simulink model "DemoUSRPTXBernoulli"  (Simulink 7.7)
settings: Solver=ode45  StartTime=0.0  StopTime=10  RelTol=1e-3
PreLoadFcn:
  | EbNo = 16; Errors = 188; Bits = 1e8; M = 256; N = 64; Ts = (1/22050); constellation; InnerInterleaverBitTable
undefined symbols (not defined in the file or in its folder): rsgenpoly
libraries: dspmtrx3 x16, simulink x9, commutil2 x3, commrandsrc2 x2, commblkintrlv2 x2, commblkcod2 x1, dspindex x1, commseqgen2 x1, commcnvintrlv2 x1, commcnvcod2 x1, dspxfrm3 x1, dspsigops x1
settings Model: Creator=katsikas  LastModifiedBy=katsikas
settings SimEventsCC: propDiagAttribOutput=1  propDiagFcnCallOutput=1  propDiagStatOutput=0

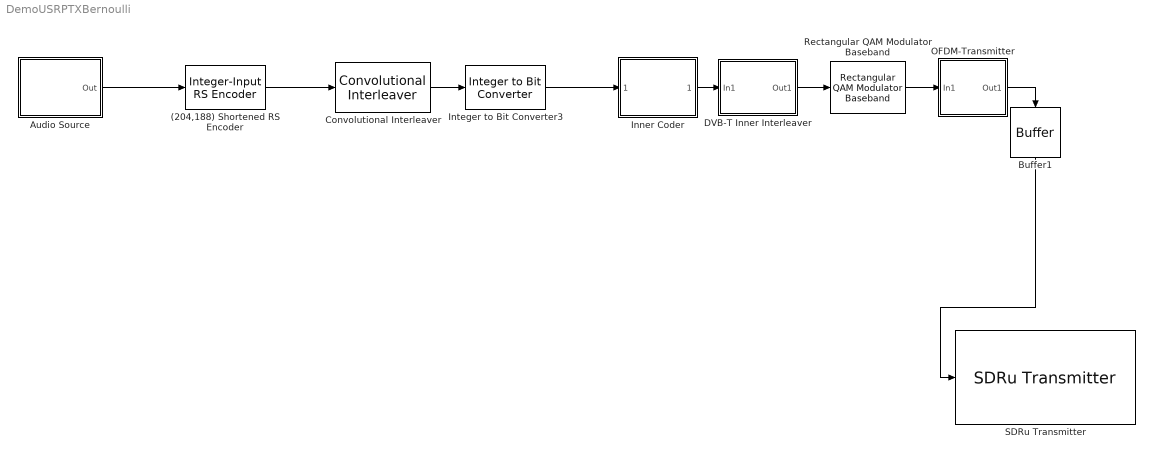
== system DemoUSRPTXBernoulli ==
  (204,188) Shortened RS Encoder : commblkcod2/Integer-Input RS Encoder  n=204  k=188  specPrimPoly=off  prPoly=[1 0 1 1]  specGenPoly=off  genPoly=rsgenpoly(7,3)  specPuncture=off  punctVec=[ones(2,1); zeros(2,1)]
  Audio Source : Subsystem
  Buffer1 : Buffer  N=2048  TreatMby1Signals=One channel
  Convolutional Interleaver : commcnvintrlv2/Convolutional Interleaver  SystemSampleTime=-1  N=12  B=17  ic=0
  DVB-T Inner Interleaver : Subsystem  mask(DVB-T Inner Interleaver){}
      mask init:
      | fullILVec = [(1:126) ...
      |  (rem([0:125]+63,126) +1 + 126     ) ...
      |  (rem([0:125]+105,126)+1 + (2*126) ) ...
      |  (rem([0:125]+42,126) +1 + (3*126) ) ...
      |  (rem([0:125]+21,126) +1 + (4*126) ) ...
      |  (rem([0:125]+84,126) +1 + (5*126) )];
      mask Display: disp('DVB-T\nInner\nInterleaver')
  Inner Coder : Subsystem
      mask Display: disp('Rate 3/4\nPunctured\nConvolutional\nCode');
  Integer to Bit Converter3 : commutil2/Integer to Bit Converter  nbits=log2(M)  signedInputValues=Unsigned  bitOrder=MSB first  outDtype=boolean
  OFDM-Transmitter : Subsystem
  Rectangular QAM Modulator Baseband : commdigbbndam3/Rectangular QAM Modulator Baseband  M=N  InType=Bit  Enc=User-defined  Mapping=map_constellation  PowType=Average Power  MinDist=2  AvgPow=1  PeakPow=1  Ph=0  outDtype=double  outWordLen=16  outUDDataType=sfix(16)  outFracLenMode=Best precision  outFracLen=15
  SDRu Transmitter : commsdrhw_v2/SDRu Transmitter  SystemSampleTime=-1  rxtx=tx  USRP2_IP='192.168.10.2'  centerFrequency=482e6  centerFrequencySrc=Dialog  loOffset=0  loOffsetSrc=Dialog  gain=20  gainSrc=Dialog  decimInterp=512  decimInterpSrc=Dialog  USRP2_IP_NUM=[49 57 50 46 49 54 56 46 49 48 46 50]  frameLength=362  outputDatatype=int16  overrunUnderrunPort=off  sampleTime=1  dboardInfo=|  HOST_DATA_PORT=30000  HOST_CONTROL_PORT=30001  USRP2_DATA_PORT=32769  USRP2_CONTROL_PORT=32768
      | dbid: 0
      |           dbName: 'no db found'
      |          freqMin: 0
      |          freqMax: 0
      |          gainMin: 0
      |          gainMax: 0
      |     gainStepSize: 0
  wires:
  Rectangular QAM Modulator Baseband/1 -> OFDM-Transmitter/1(In1)
  Convolutional Interleaver/1 -> Integer to Bit Converter3/1
  (204,188) Shortened RS Encoder/1 -> Convolutional Interleaver/1
  Integer to Bit Converter3/1 -> Inner Coder/1(Uncoded symbols)
  Inner Coder/1(Coded bits) -> DVB-T Inner Interleaver/1(In1)
  DVB-T Inner Interleaver/1(Out1) -> Rectangular QAM Modulator Baseband/1
  Audio Source/1(Out) -> (204,188) Shortened RS Encoder/1
  OFDM-Transmitter/1(Out1) -> Buffer1/1
  Buffer1/1 -> SDRu Transmitter/1

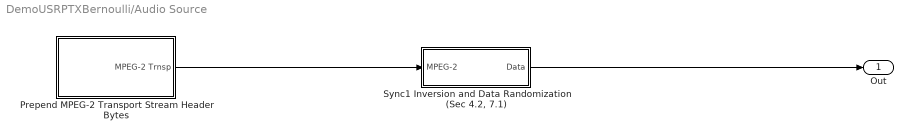
== system DemoUSRPTXBernoulli/Audio Source ==
  Prepend MPEG-2 Transport Stream Header Bytes : Subsystem
      mask Display: disp(sprintf('Prepend MPEG-2\nTransportStream\nHeader Bytes'))
  "Sync1 Inversion and Data Randomization (Sec 4.2, 7.1)" : Subsystem
  Out : Outport
  wires:
  Prepend MPEG-2 Transport Stream Header Bytes/1(MPEG-2 Trnsp) -> "Sync1 Inversion and Data Randomization (Sec 4.2, 7.1)"/1(MPEG-2)
  "Sync1 Inversion and Data Randomization (Sec 4.2, 7.1)"/1(Data) -> Out/1

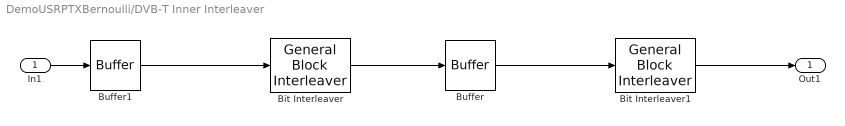
== system DemoUSRPTXBernoulli/DVB-T Inner Interleaver ==
  In1 : Inport
  Bit Interleaver : commblkintrlv2/General Block Interleaver  elements=BitInterleaverTable
  Bit Interleaver1 : commblkintrlv2/General Block Interleaver  elements=SymbolInterleaverTable
  Buffer : Buffer  N=9072  TreatMby1Signals=One channel
  Buffer1 : Buffer  N=756  TreatMby1Signals=One channel
  Out1 : Outport
  wires:
  In1/1 -> Buffer1/1
  Buffer/1 -> Bit Interleaver1/1
  Buffer1/1 -> Bit Interleaver/1
  Bit Interleaver/1 -> Buffer/1
  Bit Interleaver1/1 -> Out1/1

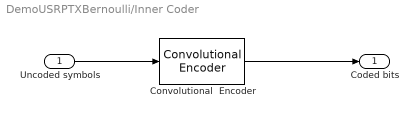
== system DemoUSRPTXBernoulli/Inner Coder ==
  Uncoded symbols : Inport
  Convolutional  Encoder : commcnvcod2/Convolutional Encoder  trellis=poly2trellis(7, [171 133])  opMode=Continuous  DelayedResetAction=off  hasIniStPort=off  hasFinStPort=off  usePuncVector=on  punctureVector=[1 1 0 1 1 0]'  reset=Unused parameter value
  Coded bits : Outport
  wires:
  Convolutional  Encoder/1 -> Coded bits/1
  Uncoded symbols/1 -> Convolutional  Encoder/1

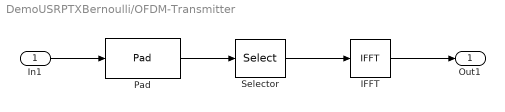
== system DemoUSRPTXBernoulli/OFDM-Transmitter ==
  In1 : Inport
  IFFT : dspxfrm3/IFFT  CompMethod=Table lookup  TableOpt=NEW  TableOptActive=Speed  BitRevOrder=off  cs_in=off  SkipNorm=on  InheritFFTLength=on  FFTLength=64  mode=Complex  outSamplingMode=Frame based  RowConvenienceOn=on  firstCoeffDataTypeStr=Inherit: Same word length as input  firstCoeffLastDataTypeStr=Inherit: Same word length as input  outputMin=[]  outputMax=[]  roundingMode=Floor  overflowMode=off
  Pad : dspsigops/Pad  padAlong=Columns  dimsToPad=1  valSrc=Specify via dialog  padVal=0  spec=Output size  padNumOutRowsSpecMethod=User-specified  numOutRows=2048  padNumOutColsSpecMethod=User-specified  numOutCols=1  isVarDimsMode=off  padBeginning=0  padEnd=0  outSizeMode=User-specified  outSize=1  padSigAt=End  trunc_flag=None  roundingMode=Floor  overflowMode=off  truncOrWrapMode=Truncate  wrap_flag=None
  Selector : Selector  NumberOfDimensions=2  InputPortWidth=3  IndexOptions=Index vector (dialog),Select all  Indices=[1:756 1513:2048 757:1512],1  OutputSizes=1,1
  Out1 : Outport
  wires:
  Pad/1 -> Selector/1
  Selector/1 -> IFFT/1
  IFFT/1 -> Out1/1
  In1/1 -> Pad/1

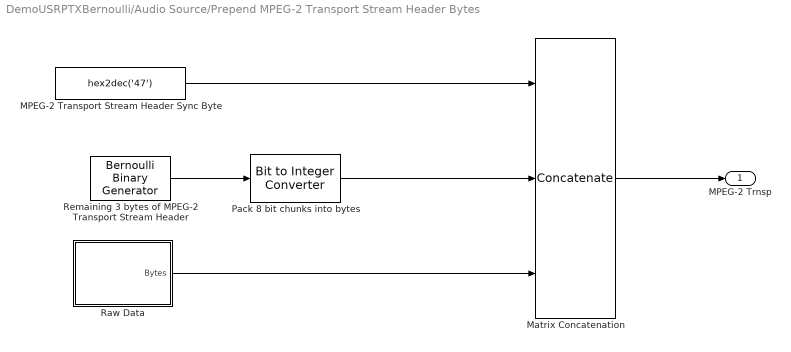
== system DemoUSRPTXBernoulli/Audio Source/Prepend MPEG-2 Transport Stream Header Bytes ==
  MPEG-2 Transport Stream Header Sync Byte : Constant  Value=hex2dec('47')  VectorParams1D=off  OutDataTypeStr=uint8  FramePeriod=(8*188)/9.6e6
      settings: SamplingMode=Frame based
  Matrix Concatenation : Concatenate  NumInputs=3  Mode=Multidimensional array
  Pack 8 bit chunks into bytes : commutil2/Bit to Integer Converter  nbits=8  bitOrder=MSB first  signedOutputValues=Unsigned  outDtype=uint8  outDtypeSigned=Inherit via internal rule
  "Raw Data " : Subsystem
  Remaining 3 bytes of MPEG-2 Transport Stream Header : commrandsrc2/Bernoulli Binary Generator  SystemSampleTime=-1  P=0.5  seed=61  Ts=(8*188/9.6e6) / (3*8)  frameBased=on  sampPerFrame=3*8  orient=off  outDataType=uint8
  MPEG-2 Trnsp : Outport
  wires:
  MPEG-2 Transport Stream Header Sync Byte/1 -> Matrix Concatenation/1
  Remaining 3 bytes of MPEG-2 Transport Stream Header/1 -> Pack 8 bit chunks into bytes/1
  Matrix Concatenation/1 -> MPEG-2 Trnsp/1
  Pack 8 bit chunks into bytes/1 -> Matrix Concatenation/2
  "Raw Data "/1(Bytes) -> Matrix Concatenation/3

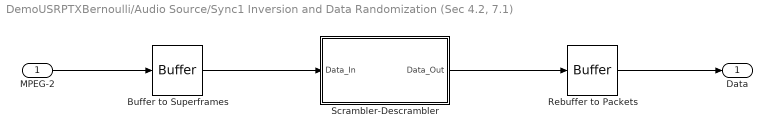
== system DemoUSRPTXBernoulli/Audio Source/Sync1 Inversion and Data Randomization (Sec 4.2, 7.1) ==
  MPEG-2 : Inport
  Buffer to Superframes : Buffer  N=1504  TreatMby1Signals=One channel
  Rebuffer to Packets : Buffer  N=188  TreatMby1Signals=One channel
  Scrambler-Descrambler : Subsystem
  Data : Outport
  wires:
  MPEG-2/1 -> Buffer to Superframes/1
  Rebuffer to Packets/1 -> Data/1
  Buffer to Superframes/1 -> Scrambler-Descrambler/1(Data_In)
  Scrambler-Descrambler/1(Data_Out) -> Rebuffer to Packets/1

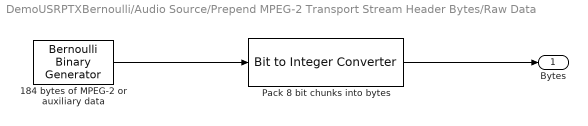
== system DemoUSRPTXBernoulli/Audio Source/Prepend MPEG-2 Transport Stream Header Bytes/Raw Data  ==
  184 bytes of MPEG-2 or auxiliary data : commrandsrc2/Bernoulli Binary Generator  SystemSampleTime=-1  P=0.5  seed=61  Ts=(8*188/9.6e6)/ (8 * 184)  frameBased=on  sampPerFrame=8 * 184  orient=off  outDataType=uint8
  Pack 8 bit chunks into bytes : commutil2/Bit to Integer Converter  nbits=8  bitOrder=MSB first  signedOutputValues=Unsigned  outDtype=uint8  outDtypeSigned=Inherit via internal rule
  Bytes : Outport
  wires:
  184 bytes of MPEG-2 or auxiliary data/1 -> Pack 8 bit chunks into bytes/1
  Pack 8 bit chunks into bytes/1 -> Bytes/1

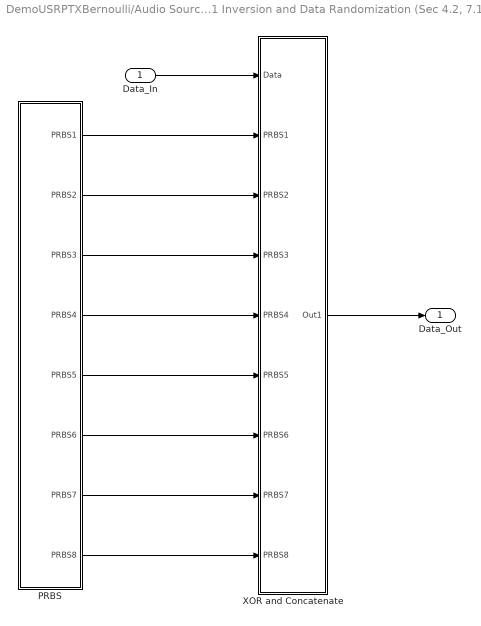
== system DemoUSRPTXBernoulli/Audio Source/Sync1 Inversion and Data Randomization (Sec 4.2, 7.1)/Scrambler-Descrambler ==
  Data_In : Inport
  PRBS : Subsystem
  XOR and Concatenate : Subsystem
  Data_Out : Outport
  wires:
  PRBS/1(PRBS1) -> XOR and Concatenate/2(PRBS1)
  PRBS/2(PRBS2) -> XOR and Concatenate/3(PRBS2)
  PRBS/3(PRBS3) -> XOR and Concatenate/4(PRBS3)
  PRBS/4(PRBS4) -> XOR and Concatenate/5(PRBS4)
  PRBS/5(PRBS5) -> XOR and Concatenate/6(PRBS5)
  PRBS/6(PRBS6) -> XOR and Concatenate/7(PRBS6)
  PRBS/7(PRBS7) -> XOR and Concatenate/8(PRBS7)
  PRBS/8(PRBS8) -> XOR and Concatenate/9(PRBS8)
  Data_In/1 -> XOR and Concatenate/1(Data)
  XOR and Concatenate/1(Out1) -> Data_Out/1

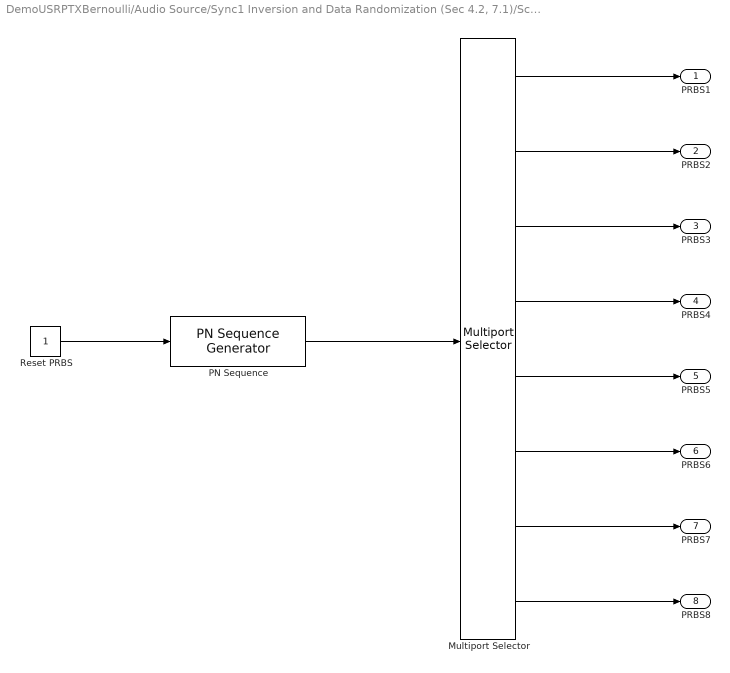
== system DemoUSRPTXBernoulli/Audio Source/Sync1 Inversion and Data Randomization (Sec 4.2, 7.1)/Scrambler-Descrambler/PRBS ==
  Multiport Selector : dspindex/Multiport Selector  rowsOrCols=Rows  idxCellArray={[1:187], [189:375], [377:563], [565:751], [753:939], [941:1127], [1129:1315], [1317:1503]}  idxErrMode=Clip Index
  PN Sequence : commseqgen2/PN Sequence Generator  poly=[15 1 0]  ini_sta=[1 0 0 1 0 1 0 1 0 0 0 0 0 0 0]  outBitMaskSource=Dialog parameter  shift=15  outVarSiz=off  maxOutSizeMode=Dialog parameter  maxOutSize=[10 1]  Ts=8 * (8*188/9.6e6) / (8*188 - 1)  frameBased=on  sampPerFrame=(8*188 - 1)  reset=on  bitPackedOutputs=on  outDataType=Smallest unsigned integer  numPackedBits=8  bitPackDataSigned=off  bitPackedOutDType=Smallest integer
  Reset PRBS : Constant  VectorParams1D=off  OutDataTypeStr=boolean  SampleTime=8 * (8*188/9.6e6)
  PRBS1 : Outport
  PRBS2 : Outport  Port=2
  PRBS3 : Outport  Port=3
  PRBS4 : Outport  Port=4
  PRBS5 : Outport  Port=5
  PRBS6 : Outport  Port=6
  PRBS7 : Outport  Port=7
  PRBS8 : Outport  Port=8
  wires:
  PN Sequence/1 -> Multiport Selector/1
  Multiport Selector/1 -> PRBS1/1
  Multiport Selector/2 -> PRBS2/1
  Multiport Selector/3 -> PRBS3/1
  Multiport Selector/4 -> PRBS4/1
  Multiport Selector/5 -> PRBS5/1
  Multiport Selector/6 -> PRBS6/1
  Multiport Selector/7 -> PRBS7/1
  Multiport Selector/8 -> PRBS8/1
  Reset PRBS/1 -> PN Sequence/1

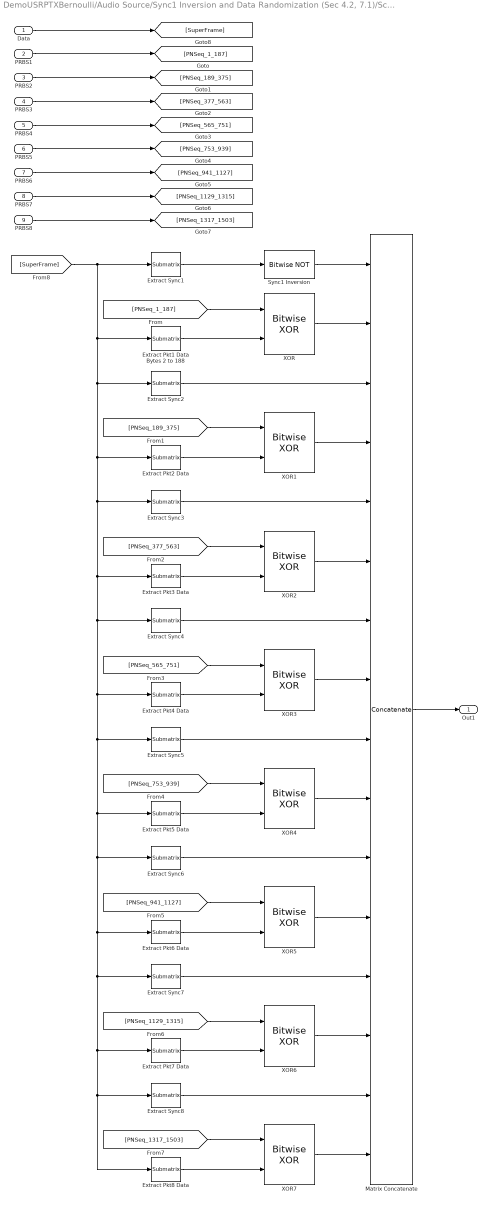
== system DemoUSRPTXBernoulli/Audio Source/Sync1 Inversion and Data Randomization (Sec 4.2, 7.1)/Scrambler-Descrambler/XOR and Concatenate ==
  Data : Inport
  PRBS1 : Inport  Port=2
  PRBS2 : Inport  Port=3
  PRBS3 : Inport  Port=4
  PRBS4 : Inport  Port=5
  PRBS5 : Inport  Port=6
  PRBS6 : Inport  Port=7
  PRBS7 : Inport  Port=8
  PRBS8 : Inport  Port=9
  Extract Pkt1 Data Bytes 2 to 188 : dspmtrx3/Submatrix  RowSpan=Range of rows  RowStartMode=Index  RowStartIndex=2  RowEndMode=Index  RowEndIndex=188  ColSpan=All columns  ColStartMode=First  ColStartIndex=1  ColEndMode=Last  ColEndIndex=1
  Extract Pkt2 Data : dspmtrx3/Submatrix  RowSpan=Range of rows  RowStartMode=Index  RowStartIndex=188+2  RowEndMode=Index  RowEndIndex=2*188  ColSpan=All columns  ColStartMode=First  ColStartIndex=1  ColEndMode=Last  ColEndIndex=1
  Extract Pkt3 Data : dspmtrx3/Submatrix  RowSpan=Range of rows  RowStartMode=Index  RowStartIndex=2*188+2  RowEndMode=Index  RowEndIndex=3*188  ColSpan=All columns  ColStartMode=First  ColStartIndex=1  ColEndMode=Last  ColEndIndex=1
  Extract Pkt4 Data : dspmtrx3/Submatrix  RowSpan=Range of rows  RowStartMode=Index  RowStartIndex=3*188+2  RowEndMode=Index  RowEndIndex=4*188  ColSpan=All columns  ColStartMode=First  ColStartIndex=1  ColEndMode=Last  ColEndIndex=1
  Extract Pkt5 Data : dspmtrx3/Submatrix  RowSpan=Range of rows  RowStartMode=Index  RowStartIndex=4*188+2  RowEndMode=Index  RowEndIndex=5*188  ColSpan=All columns  ColStartMode=First  ColStartIndex=1  ColEndMode=Last  ColEndIndex=1
  Extract Pkt6 Data : dspmtrx3/Submatrix  RowSpan=Range of rows  RowStartMode=Index  RowStartIndex=5*188+2  RowEndMode=Index  RowEndIndex=6*188  ColSpan=All columns  ColStartMode=First  ColStartIndex=1  ColEndMode=Last  ColEndIndex=1
  Extract Pkt7 Data : dspmtrx3/Submatrix  RowSpan=Range of rows  RowStartMode=Index  RowStartIndex=6*188+2  RowEndMode=Index  RowEndIndex=7*188  ColSpan=All columns  ColStartMode=First  ColStartIndex=1  ColEndMode=Last  ColEndIndex=1
  Extract Pkt8 Data : dspmtrx3/Submatrix  RowSpan=Range of rows  RowStartMode=Index  RowStartIndex=7*188+2  RowEndMode=Last  RowEndIndex=8*188  ColSpan=All columns  ColStartMode=First  ColStartIndex=1  ColEndMode=Last  ColEndIndex=1
  Extract Sync1 : dspmtrx3/Submatrix  RowSpan=One row  RowStartMode=First  RowStartIndex=1  RowEndMode=Index  RowEndIndex=8  ColSpan=All columns  ColStartMode=First  ColStartIndex=1  ColEndMode=Last  ColEndIndex=1
  Extract Sync2 : dspmtrx3/Submatrix  RowSpan=One row  RowStartMode=Index  RowStartIndex=188+1  RowEndMode=Index  RowEndIndex=8  ColSpan=All columns  ColStartMode=First  ColStartIndex=1  ColEndMode=Last  ColEndIndex=1
  Extract Sync3 : dspmtrx3/Submatrix  RowSpan=One row  RowStartMode=Index  RowStartIndex=2*188+1  RowEndMode=Index  RowEndIndex=8  ColSpan=All columns  ColStartMode=First  ColStartIndex=1  ColEndMode=Last  ColEndIndex=1
  Extract Sync4 : dspmtrx3/Submatrix  RowSpan=One row  RowStartMode=Index  RowStartIndex=3*188+1  RowEndMode=Index  RowEndIndex=8  ColSpan=All columns  ColStartMode=First  ColStartIndex=1  ColEndMode=Last  ColEndIndex=1
  Extract Sync5 : dspmtrx3/Submatrix  RowSpan=One row  RowStartMode=Index  RowStartIndex=4*188+1  RowEndMode=Index  RowEndIndex=8  ColSpan=All columns  ColStartMode=First  ColStartIndex=1  ColEndMode=Last  ColEndIndex=1
  Extract Sync6 : dspmtrx3/Submatrix  RowSpan=One row  RowStartMode=Index  RowStartIndex=5*188+1  RowEndMode=Index  RowEndIndex=8  ColSpan=All columns  ColStartMode=First  ColStartIndex=1  ColEndMode=Last  ColEndIndex=1
  Extract Sync7 : dspmtrx3/Submatrix  RowSpan=One row  RowStartMode=Index  RowStartIndex=6*188+1  RowEndMode=Index  RowEndIndex=8  ColSpan=All columns  ColStartMode=First  ColStartIndex=1  ColEndMode=Last  ColEndIndex=1
  Extract Sync8 : dspmtrx3/Submatrix  RowSpan=One row  RowStartMode=Index  RowStartIndex=7*188+1  RowEndMode=Index  RowEndIndex=8  ColSpan=All columns  ColStartMode=First  ColStartIndex=1  ColEndMode=Last  ColEndIndex=1
  Matrix Concatenate : Concatenate  NumInputs=16  Mode=Multidimensional array
  Sync1 Inversion : simulink/Logic and Bit Operations/Bitwise Operator  logicop=NOT  UseBitMask=off  BitMask=bin2dec('11011001')  BitMaskRealWorld=Stored Integer
  XOR{,1..7} (8 alike) : simulink/Logic and Bit Operations/Bitwise Operator  logicop=XOR  UseBitMask=off  NumInputPorts=2  BitMask=bin2dec('11011001')  BitMaskRealWorld=Stored Integer
  Out1 : Outport
  wires:
  [SuperFrame] -> Extract Pkt2 Data/1, Extract Pkt3 Data/1, Extract Pkt4 Data/1, Extract Pkt5 Data/1, Extract Pkt6 Data/1, Extract Pkt8 Data/1, Extract Sync8/1, Extract Pkt7 Data/1, Extract Sync7/1, Extract Sync6/1, Extract Sync5/1, Extract Sync4/1, Extract Sync3/1, Extract Sync2/1, Extract Pkt1 Data Bytes 2 to 188/1, Extract Sync1/1
  Extract Sync1/1 -> Sync1 Inversion/1
  Extract Pkt1 Data Bytes 2 to 188/1 -> XOR/2
  [PNSeq_1_187] -> XOR/1
  Sync1 Inversion/1 -> Matrix Concatenate/1
  XOR/1 -> Matrix Concatenate/2
  Extract Sync2/1 -> Matrix Concatenate/3
  Extract Sync3/1 -> Matrix Concatenate/5
  Extract Sync4/1 -> Matrix Concatenate/7
  Extract Sync5/1 -> Matrix Concatenate/9
  Extract Sync6/1 -> Matrix Concatenate/11
  Extract Sync7/1 -> Matrix Concatenate/13
  Extract Sync8/1 -> Matrix Concatenate/15
  XOR1/1 -> Matrix Concatenate/4
  XOR2/1 -> Matrix Concatenate/6
  XOR3/1 -> Matrix Concatenate/8
  XOR4/1 -> Matrix Concatenate/10
  XOR5/1 -> Matrix Concatenate/12
  XOR6/1 -> Matrix Concatenate/14
  XOR7/1 -> Matrix Concatenate/16
  [PNSeq_189_375] -> XOR1/1
  [PNSeq_377_563] -> XOR2/1
  [PNSeq_565_751] -> XOR3/1
  [PNSeq_753_939] -> XOR4/1
  [PNSeq_941_1127] -> XOR5/1
  [PNSeq_1129_1315] -> XOR6/1
  [PNSeq_1317_1503] -> XOR7/1
  Extract Pkt2 Data/1 -> XOR1/2
  Extract Pkt3 Data/1 -> XOR2/2
  Extract Pkt4 Data/1 -> XOR3/2
  Extract Pkt5 Data/1 -> XOR4/2
  Extract Pkt6 Data/1 -> XOR5/2
  Extract Pkt7 Data/1 -> XOR6/2
  Extract Pkt8 Data/1 -> XOR7/2
  Matrix Concatenate/1 -> Out1/1
  PRBS1/1 -> [PNSeq_1_187]
  PRBS2/1 -> [PNSeq_189_375]
  PRBS3/1 -> [PNSeq_377_563]
  PRBS4/1 -> [PNSeq_565_751]
  PRBS5/1 -> [PNSeq_753_939]
  PRBS6/1 -> [PNSeq_941_1127]
  PRBS7/1 -> [PNSeq_1129_1315]
  PRBS8/1 -> [PNSeq_1317_1503]
  Data/1 -> [SuperFrame]
